simulink model "sgMdl_IO135_IO316_InterModuleSyncLoopback"  (R2024b)
settings: Solver=FixedStepAuto  StartTime=0.0  StopTime=inf  RelTol=1e-3
undefined symbols (not defined in the file): IO132, IO135, IO316, Pull, pull, up
libraries: speedgoatlib_IO135 x2, speedgoatlib_fpga_pwm x1, speedgoatlib_fpga x1, speedgoatlib_interrupt x1
Description:
  | IO135 - IO316 Inter-Module Synchronization Loopback
settings Model: ModifiedByFormat=Speedgoat  SimulationMode=external  ExtModeTrigDuration=100000  Creator=Speedgoat  LastModifiedBy=Speedgoat
settings SolverCC: ConcurrentTasks=on  PositivePriorityOrder=on
settings DataIOCC: SaveFormat=StructureWithTime
settings OptimizationCC: BlockReduction=off  OptimizeBlockIOStorage=off  BufferReuse=off
settings DebuggingCC: UnderspecifiedInitializationDetection=Classic  MergeDetectMultiDrivingBlocksExec=none  TasksWithSamePriorityMsg=none
settings HardwareCC: ProdBitPerLong=64  ProdLongLongMode=on  ProdHWDeviceType=Intel->x86-64 (Linux 64)
settings ModelReferenceCC: EnableRefExpFcnMdlSchedulingChecks=on  PropagateSignalLabelsOutOfModel=off
settings RTWCC: Description=Speedgoat Real-Time Target Machine  SystemTargetFile=speedgoat.tlc  TemplateMakefile=slrealtime_default_tmf  PostCodeGenCommand=sg.model.build.makeCfg(bdroot, buildInfo);  Toolchain=Simulink Real-Time Toolchain  BuildConfiguration=Faster Runs  TargetLang=C++  GPUComputeCapability=3.5
settings SimulinkRealTimeTargetCC: SubcomponentCodeInterfacePackaging=Reusable function  InstructionSetFMA=off  LogToMDFFile=off  SLRTFileLogMaxRuns=10
settings ConfigComp: CovBoundaryAbsTol=1.0e-5

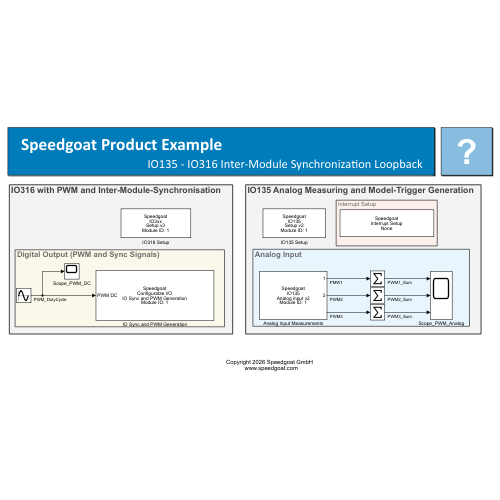
[thumbnail: Simulink's stored preview of the top-level diagram]
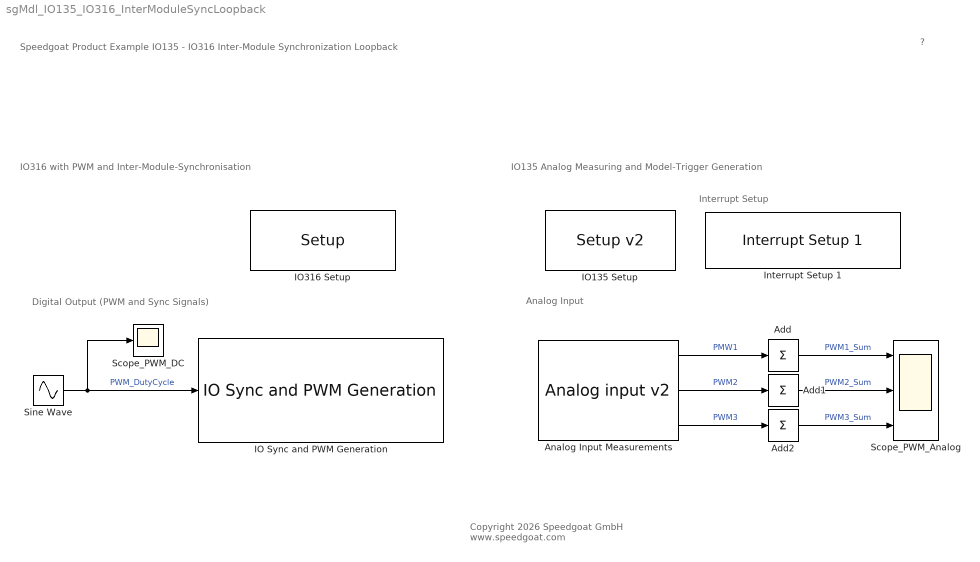
== system sgMdl_IO135_IO316_InterModuleSyncLoopback ==
  note: IO316 with PWM and Inter-Module-Synchronisation
  note: Digital Output (PWM and Sync Signals)
  note: IO135 Analog Measuring and Model-Trigger Generation
  note: Interrupt Setup
  note: Analog Input
  note: Speedgoat Product Example
      | IO135 - IO316 Inter-Module Synchronization Loopback
  note: ?
  note: Copyright 2026 Speedgoat GmbH
      |  www.speedgoat.com
  Add : Sum  Inputs=+
  Add1 : Sum  Inputs=+
  Add2 : Sum  Inputs=+
  Analog Input Measurements : speedgoatlib_IO135/Analog input v2   parModuleId=1  parSampleTime=-1  parPciSlot=-1  parAdcChannels=[1 9 17]  parAdcVoltageRange=[1 1 1 1]  parAdcOversamplRate=[1 1 1 1]  parAdcContSampling=0  parAdcDmaEnable=1  parAdcActiveDmaDevices=[1 1 1 1]  parAdcFrameSize=1000
      settings: SourceProductName=Simulink Real-Time: Speedgoat I/O Blockset
  IO Sync and PWM Generation : speedgoatlib_fpga_pwm/IO Sync and PWM Generation  id=1  channelVector=[1:8]  channelSelectionDropdown=3  ts=-1  basePwmPeriod=10e-3  actualBasePwmPeriod=0.010000000000000000208  dutyCycleAlignment=Right-aligned  deadbandScalar=0  pwm_update=At period starts  ioModuleFamily=IO132-IO135  IO106_sampleMode=Single sample per period  IO106_Single_SamplePosition=Start of base PWM period  numberOfSamplesIO106=1  IO13x_sampleMode=Multiple samples per period  IO3x_Single_SamplePosition=Start of base PWM period  numberOfSamplesIO13x=1000  IO13x_frameTriggerPosition=1  trigger_period_start=on  trigger_half_of_the_period=off  trigger_a_on=off  trigger_a_off=off  trigger_b_on=off  trigger_b_off=off
      link override PWM generation: pciSlot=-1
      link override PWM generation1: pciSlot=-1
      settings: SourceProductName=Simulink Real-Time: Speedgoat I/O Blockset
  IO135 Setup : speedgoatlib_IO135/Setup v2   parPciSlot=-1  parModuleId=1  parInterModuleSync=Target - Rear I/O  parConvClockBaseRate=20MHz  parConvClock1Divider=200  parConvClock2Divider=200  parFrameTriggerEnable=on  parFrameTriggerDivider=1000  parConvClock1BaseRate=1  parConvClock2BaseRate=1  parFrameTriggerClock=1  parAdcChannels=[1 9 17]  parAdcRange1=+-5V  parAdcRange2=+-5V  parAdcRange3=+-5V  parAdcRange4=+-5V  parAdcVoltageRange=[1 1 1 1]  parAdcOversampling1=None  parAdcOversampling2=None  parAdcOversampling3=None  parAdcOversampling4=None  parAdcOversamplRate=[1 1 1 1]  parAdcContSampling=off  parAdcDataCorrection=Automatic  parAdcCorrectionActive={}  parAdcCorrectionPm5V={'1','0','0';'2','0','0';'3','0','0';'4','0','0';'5','0','0';'6','0','0';'7','0','0';'8','0','0';'9','0','0';'10','0','0';'11','0','0';'12','0','0';'13','0','0';'14','0',' 0';'15','0','0';'16','0','0';'17','0','0';'18','0','0';'19','0','0';'20','0','0';'21','0','0';'22','0','0';'23','0','0';'24','0','0';'25','0','0';'26','0','0';'27','0','0';'28','0','0';'29','0','0';'30','0','0';'31','0','0';'32','0','0'}  parAdcCorrectionPm10V={'1','0','0';'2','0','0';'3','0','0';'4','0','0';'5','0','0';'6','0','0';'7','0','0';'8','0','0';'9','0','0';'10','0','0';'11','0','0';'12','0','0';'13','0','0';'14','0',' 0';'15','0','0';'16','0','0';'17','0','0';'18','0','0';'19','0','0';'20','0','0';'21','0','0';'22','0','0';'23','0','0';'24','0','0';'25','0','0';'26','0','0';'27','0','0';'28','0','0';'29','0','0';'30','0','0';'31','0','0';'32','0','0'}  parAdcDmaEnable=on  parAdcDmaClock=Clock 1  parAdcFrameSize_=1000  parAdcSampleTime_=-1  parAdcActiveDmaDevices=[1 1 1 1]  parAdcFrameTriggerEnable=1  parAdcFrameSize=1000  parAdcSampleTime=0.01  parDacChannels=[1 2]  parDacInitValues=0  parDacReset=1  parDacRange1=0-5V  parDacRange2=0-5V  parDacRange3=0-5V  parDacRange4=0-5V  parDacRange5=0-5V  parDacRange6=0-5V  parDacRange7=0-5V  parDacRange8=0-5V  parDacRange9=0-5V  parDacRange10=0-5V  parDacRange11=0-5V  parDacRange12=0-5V  parDacRange13=0-5V  parDacRange14=0-5V  parDacRange15=0-5V  parDacRange16=0-5V  parDacVoltageRange=[1 1 1 1 1 1 1 1 1 1 1 1 1 1 1 1]  parDacSyncOut=on  parDacDataCorrection=Automatic  parDacCorrectionActive={}  parDacCorrection5V={'1','0','0';'2','0','0';'3','0','0';'4','0','0';'5','0','0';'6','0','0';'7','0','0';'8','0','0';'9','0','0';'10','0','0';'11','0','0';'12','0','0';'13','0','0';'14','0',' 0';'15','0','0';'16','0','0'}  parDacCorrection10V={'1','0','0';'2','0','0';'3','0','0';'4','0','0';'5','0','0';'6','0','0';'7','0','0';'8','0','0';'9','0','0';'10','0','0';'11','0','0';'12','0','0';'13','0','0';'14','0',' 0';'15','0','0';'16','0','0'}  parDacCorrection10_8V={'1','0','0';'2','0','0';'3','0','0';'4','0','0';'5','0','0';'6','0','0';'7','0','0';'8','0','0';'9','0','0';'10','0','0';'11','0','0';'12','0','0';'13','0','0';'14','0',' 0';'15','0','0';'16','0','0'}  parDacCorrectionPm5V={'1','0','0';'2','0','0';'3','0','0';'4','0','0';'5','0','0';'6','0','0';'7','0','0';'8','0','0';'9','0','0';'10','0','0';'11','0','0';'12','0','0';'13','0','0';'14','0',' 0';'15','0','0';'16','0','0'}  parDacCorrectionPm10V={'1','0','0';'2','0','0';'3','0','0';'4','0','0';'5','0','0';'6','0','0';'7','0','0';'8','0','0';'9','0','0';'10','0','0';'11','0','0';'12','0','0';'13','0','0';'14','0',' 0';'15','0','0';'16','0','0'}  parDacCorrectionPm10_8V={'1','0','0';'2','0','0';'3','0','0';'4','0','0';'5','0','0';'6','0','0';'7','0','0';'8','0','0';'9','0','0';'10','0','0';'11','0','0';'12','0','0';'13','0','0';'14','0',' 0';'15','0','0';'16','0','0'}  parDacDmaEnable=off  parDacDmaLatency=Until next frame  parDacDmaClock=Clock 1  parDacFrameSize_=100  parDacSampleTime_=-1  parDacActiveDmaDevices=[1 1 1 1]  parDacFrameTriggerEnable=1  parDacFrameSize=100  parDacSampleTime=0.001  parDoChannels=[1 2]  parDoInitValues=0  parDoReset=1  parDiChannels=[3 4]  parDiDebounceEnable=off  parDiDebounceTime=0  parDiDebounceValue=0  parDioPullRefFront=Pull-up 3.3V  parDioPullRefRear=Floating
      settings: SourceProductName=Simulink Real-Time: Speedgoat I/O Blockset
  IO316 Setup : speedgoatlib_fpga/Setup/Setup  board=IO316-100k  id=1  pciSlot=-1  device_id=1  bitstreamFilePath=[]  bitstreamFile=speedgoat_IO316_100k_IO13xSync_test.mat  fpgaFreq=75 MHz  enableDma=off  rearEnb_1=off  rearIO_1=None  rearEnb_2=off  rearIO_2=None  ProgSpiFlash=off  ProgBPIFlash=off  useFpgaDmaController=off  dmaTrigDropdown=Model Step  dmaTrigSelect=0  dmaStopOnOverload=on  dmaModeSequential=on  dmaModeParallel=off  PullRPort15=pull-up 3.3V  PullRPort31=pull-up 3.3V  PullRPort47=pull-up 3.3V  PullRPort63=pull-up 3.3V  diffLineTermination_1=on  diffLineTermination_2=on  diffLineTermination_3=on  diffLineTermination_4=on  diffLineTermination_5=on  diffLineTermination_6=on  diffLineTermination_7=on  diffLineTermination_8=on  diffLineTermination_9=on  diffLineTermination_10=on  diffLineTermination_11=on  diffLineTermination_12=on  diffLineTermination_13=on  diffLineTermination_14=on  diffLineTermination_15=on  diffLineTermination_16=on  diffLineTermination_17=on  diffLineTermination_18=on  diffLineTermination_19=on  diffLineTermination_20=on  diffLineTermination_21=on  diffLineTermination_22=on  diffLineTermination_23=on  diffLineTermination_24=on  diffLineTermination_25=on  diffLineTermination_26=on  diffLineTermination_27=on  diffLineTermination_28=on  diffLineTermination_29=on  diffLineTermination_30=on  diffLineTermination_31=on  diffLineTermination_32=on  ioVoltageDropDown1=3.3V  pullResistorDropDown1_1=Pull-up  pullResistorDropDown1_2=Pull-up  pullResistorDropDown1_3=Pull-up  pullResistorDropDown1_4=Pull-up  pullResistorDropDown1_5=Pull-up  pullResistorDropDown1_6=Pull-up  pullResistorDropDown1_7=Pull-up  pullResistorDropDown1_8=Pull-up  ttlIsImplementedCheckBox1=off  pullResistorDropDown2=Pull-up  ioVoltageDropDown2=3.3V  ttlIsImplementedCheckBox2=off  pullResistorDropDown3=Pull-up  ioVoltageDropDown3=3.3V  ttlIsImplementedCheckBox3=off  pullResistorDropDown4=Pull-up  ioVoltageDropDown4=3.3V  ttlIsImplementedCheckBox4=off  pullResistorDropDown5=Pull-up  ioVoltageDropDown5=3.3V  ttlIsImplementedCheckBox5=off  pullResistorDropDown6=Pull-up  ioVoltageDropDown6=3.3V  ttlIsImplementedCheckBox6=off  pullResistorDropDown7=Pull-up  ioVoltageDropDown7=3.3V  ttlIsImplementedCheckBox7=off  pullResistorDropDown8=Pull-up  ioVoltageDropDown8=3.3V  ttlIsImplementedCheckBox8=off  terminationCheckBox1=off  terminationCheckBox2=off  terminationCheckBox3=off  terminationCheckBox4=off  diffIsImplementedCheckBox1=off  terminationCheckBox5=off  terminationCheckBox6=off  terminationCheckBox7=off  terminationCheckBox8=off  diffIsImplementedCheckBox2=off  terminationCheckBox9=off  terminationCheckBox10=off  terminationCheckBox11=off  terminationCheckBox12=off  diffIsImplementedCheckBox3=off  terminationCheckBox13=off  terminationCheckBox14=off  terminationCheckBox15=off  terminationCheckBox16=off  diffIsImplementedCheckBox4=off  terminationCheckBox17=off  terminationCheckBox18=off  terminationCheckBox19=off  terminationCheckBox20=off  diffIsImplementedCheckBox5=off  terminationCheckBox21=off  terminationCheckBox22=off  terminationCheckBox23=off  terminationCheckBox24=off  diffIsImplementedCheckBox6=off  terminationCheckBox25=off  terminationCheckBox26=off  terminationCheckBox27=off  terminationCheckBox28=off  diffIsImplementedCheckBox7=off  terminationCheckBox29=off  terminationCheckBox30=off  terminationCheckBox31=off  terminationCheckBox32=off  diffIsImplementedCheckBox8=off  PullRPort0_1=pull-up  VioPort0_1=3.3V  PullRPort1_1=pull-up  VioPort1_1=3.3V  PullRPort2_1=pull-up  VioPort2_1=3.3V  PullRPort3_1=pull-up  VioPort3_1=3.3V  PullRPort4_1=pull-up  VioPort4_1=3.3V  PullRPort5_1=pull-up  VioPort5_1=3.3V  PullRPort6_1=pull-up  VioPort6_1=3.3V  diffLineTermination_rear1_1=on  diffLineTermination_rear1_2=on  diffLineTermination_rear1_3=on  diffLineTermination_rear1_4=on  diffLineTermination_rear1_5=on  diffLineTermination_rear1_6=on  diffLineTermination_rear1_7=on  diffLineTermination_rear1_8=on  PullRPort0_2=pull-up  VioPort0_2=3.3V  PullRPort1_2=pull-up  VioPort1_2=3.3V  PullRPort2_2=pull-up  VioPort2_2=3.3V  PullRPort3_2=pull-up  VioPort3_2=3.3V  PullRPort4_2=pull-up  VioPort4_2=3.3V  PullRPort5_2=pull-up  VioPort5_2=3.3V  PullRPort6_2=pull-up  VioPort6_2=3.3V  diffLineTermination_rear2_1=on  diffLineTermination_rear2_2=on  diffLineTermination_rear2_3=on  diffLineTermination_rear2_4=on  diffLineTermination_rear2_5=on  diffLineTermination_rear2_6=on  diffLineTermination_rear2_7=on  diffLineTermination_rear2_8=on
      settings: SourceProductName=Simulink Real-Time: Speedgoat I/O Blockset
  Interrupt Setup 1 : speedgoatlib_interrupt/Interrupt Setup 1  parModuleTrigger=on  parPollingMode=off  parPriorityConf=High  parPriority=241  confStartFcn=IO135_start_public  confStopFcn=IO135_stop_public  confIsrFcn=IO135_isr_public  confMapFcn=IO135_map_public  confHookFile=io135_int_hooks.c  confIrqNr=-1  confIsPolling=off  confModID=16776961  confSelectedInt=Speedgoat IO135 DMA interrupt  confSelectedId=1  confSelectedChannel=[]  confData=[]  confForcePollingMode=off
  Scope_PWM_Analog : Scope  NumInputPorts=3
  Scope_PWM_DC : Scope
  Sine Wave : Sin  Amplitude=.5  Bias=.5  Frequency=2*pi/5  Phase=[0 4/3*pi 2/3*pi]  Samples=500
  wires:
  Sine Wave/1 -> IO Sync and PWM Generation/1, Scope_PWM_DC/1  "PWM_DutyCycle"
  Add/1 -> Scope_PWM_Analog/1  "PWM1_Sum"
  Add2/1 -> Scope_PWM_Analog/3  "PWM3_Sum"
  Analog Input Measurements/3 -> Add2/1  "PWM3"
  Analog Input Measurements/1 -> Add/1  "PMW1"
  Add1/1 -> Scope_PWM_Analog/2  "PWM2_Sum"
  Analog Input Measurements/2 -> Add1/1  "PWM2"
